simulink model "model"  (R2019b)
settings: Solver=VariableStepAuto  StartTime=0.0  StopTime=2  FixedStep=0.001  RelTol=1e-3
values from neighbouring files (symbols this model uses):
  b = 0.002953    [params.m]
  c = 1.25    [params.m]
  I = 0.0221    [params.m]
  K_d_m = 2.85    [params.m]
  K_d_o = 1.6    [params.m]
  K_d_zn = 1.08    [params.m]
  K_i_m = 60    [params.m]
  K_i_o = 614.4    [params.m]
  K_i_zn = 1105.92    [params.m]
  K_p_m = 103.5    [params.m]
  K_p_o = 38.4    [params.m]
  K_p_zn = 69.12    [params.m]
  L = 0.0281    [params.m]
  N_m = 7700    [params.m]
  R = 2.581    [params.m]
settings Model: Creator=Tira  LastModifiedBy=Foxy

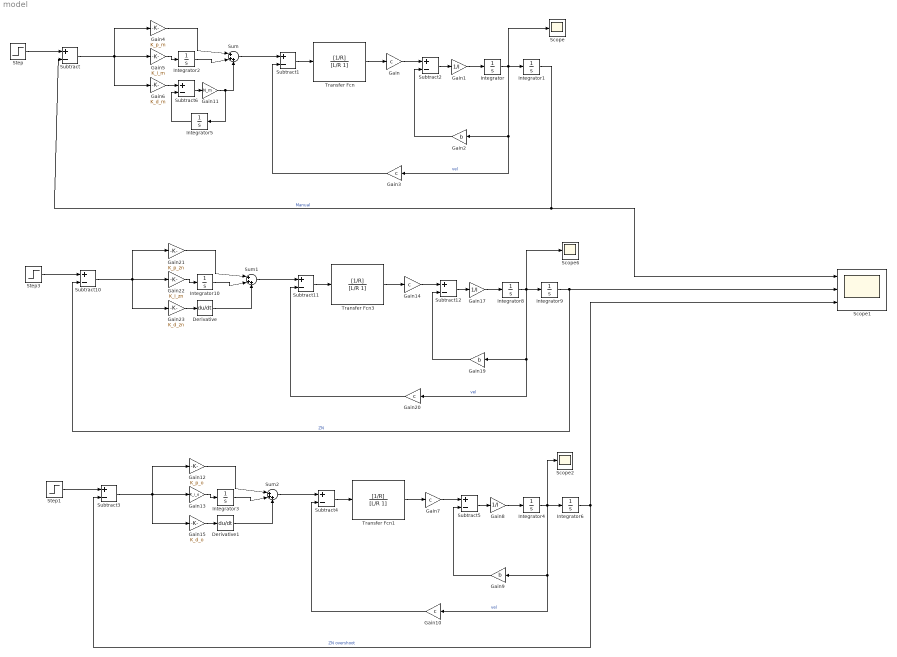
== system model ==
  Derivative : Derivative
  Derivative1 : Derivative
  Gain{,3,7,10,14,20} (6 alike) : Gain  Gain=c
  Gain1 : Gain  Gain=1/I
  Gain11 : Gain  Gain=N_m
  Gain12 : Gain  Gain=K_p_o
  Gain13 : Gain  Gain=K_i_o
  Gain15 : Gain  Gain=K_d_o
  Gain17 : Gain  Gain=1/I
  Gain19 : Gain  Gain=b
  Gain2 : Gain  Gain=b
  Gain21 : Gain  Gain=K_p_zn
  Gain22 : Gain  Gain=K_i_zn
  Gain23 : Gain  Gain=K_d_zn
  Gain4 : Gain  Gain=K_p_m
  Gain5 : Gain  Gain=K_i_m
  Gain6 : Gain  Gain=K_d_m
  Gain8 : Gain  Gain=1/I
  Gain9 : Gain  Gain=b
  Integrator{,1..6,8..10} (10 alike) : Integrator
  Scope : Scope
  Scope1 : Scope  NumInputPorts=3
  Scope2 : Scope
  Scope6 : Scope
  Step : Step  Time=0  SampleTime=0
  Step1 : Step  Time=0  SampleTime=0
  Step3 : Step  Time=0  SampleTime=0
  Subtract{,1..6,10..12} (10 alike) : Sum  Inputs=+-
  Sum : Sum  Inputs=|+++
  Sum1 : Sum  Inputs=|+++
  Sum2 : Sum  Inputs=|+++
  Transfer Fcn : TransferFcn  Numerator=[1/R]  Denominator=[L/R 1]
  Transfer Fcn1 : TransferFcn  Numerator=[1/R]  Denominator=[L/R 1]
  Transfer Fcn3 : TransferFcn  Numerator=[1/R]  Denominator=[L/R 1]
  wires:
  Gain1/1 -> Integrator/1
  Transfer Fcn/1 -> Gain/1
  Gain/1 -> Subtract2/1
  Subtract2/1 -> Gain1/1
  Integrator/1 -> Scope/1, Gain3/1, Gain2/1, Integrator1/1  "vel"
  Integrator1/1 -> Scope1/1, Subtract/2  "Manual"
  Subtract1/1 -> Transfer Fcn/1
  Sum/1 -> Subtract1/1
  Step/1 -> Subtract/1
  Subtract/1 -> Gain6/1, Gain4/1, Gain5/1
  Gain3/1 -> Subtract1/2
  Gain2/1 -> Subtract2/2
  Gain4/1 -> Sum/1
  Gain5/1 -> Integrator2/1
  Integrator2/1 -> Sum/2
  Gain11/1 -> Sum/3, Integrator5/1
  Gain6/1 -> Subtract6/1
  Subtract6/1 -> Gain11/1
  Integrator5/1 -> Subtract6/2
  Gain23/1 -> Derivative/1
  Gain19/1 -> Subtract12/2
  Gain14/1 -> Subtract12/1
  Subtract11/1 -> Transfer Fcn3/1
  Derivative/1 -> Sum1/3
  Integrator10/1 -> Sum1/2
  Gain21/1 -> Sum1/1
  Integrator8/1 -> Scope6/1, Gain20/1, Gain19/1, Integrator9/1  "vel"
  Gain22/1 -> Integrator10/1
  Step3/1 -> Subtract10/1
  Gain17/1 -> Integrator8/1
  Integrator9/1 -> Scope1/2, Subtract10/2  "ZN"
  Subtract10/1 -> Gain23/1, Gain21/1, Gain22/1
  Subtract12/1 -> Gain17/1
  Transfer Fcn3/1 -> Gain14/1
  Gain20/1 -> Subtract11/2
  Sum1/1 -> Subtract11/1
  Gain8/1 -> Integrator4/1
  Gain9/1 -> Subtract5/2
  Subtract4/1 -> Transfer Fcn1/1
  Gain10/1 -> Subtract4/2
  Transfer Fcn1/1 -> Gain7/1
  Subtract5/1 -> Gain8/1
  Gain12/1 -> Sum2/1
  Integrator4/1 -> Scope2/1, Gain10/1, Gain9/1, Integrator6/1  "vel"
  Integrator6/1 -> Scope1/3, Subtract3/2  "ZN overshoot"
  Step1/1 -> Subtract3/1
  Gain15/1 -> Derivative1/1
  Gain7/1 -> Subtract5/1
  Gain13/1 -> Integrator3/1
  Sum2/1 -> Subtract4/1
  Subtract3/1 -> Gain15/1, Gain12/1, Gain13/1
  Derivative1/1 -> Sum2/3
  Integrator3/1 -> Sum2/2
